simulink model "diff_drive"  (R2021b)
settings: Solver=VariableStepAuto  StartTime=0.0  StopTime=10.0  RelTol=1e-3
settings Model: Creator=Daniel  LastModifiedBy=Daniel

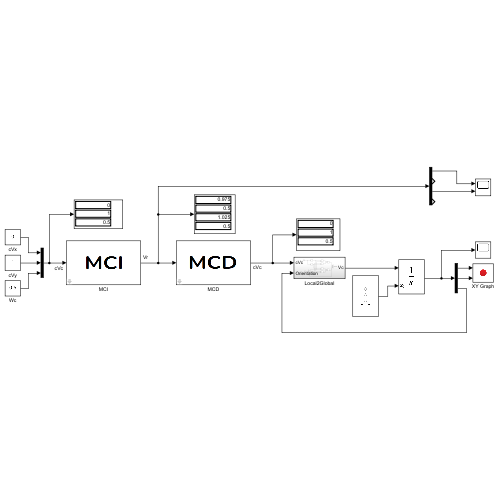
[thumbnail: Simulink's stored preview of the top-level diagram]
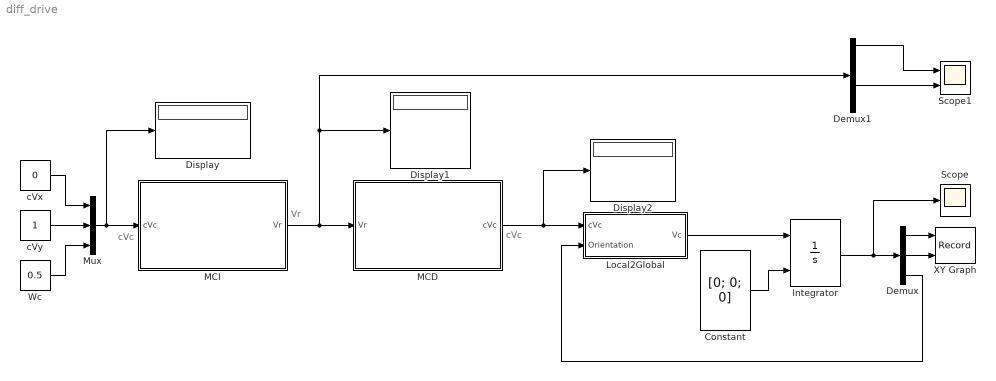
== system diff_drive ==
  note: cVc
  note: Vr
  note: cVc
  Constant : Constant  Value=[0; 0; 0]  VectorParams1D=off  SampleTime=-1
  Demux : Demux  Outputs=3
  Demux1 : Demux
  Display : Display
  Display1 : Display
  Display2 : Display
  Integrator : Integrator  InitialConditionSource=external
  Local2Global : Subsystem
  MCD : Subsystem  mask{d1=0.05, d2=0.05}
      mask prompts: d1 "Distancia del centro a la rueda 1 (m)"; d2 "Distancia del centro a la rueda 1 (m)"
      mask Display: image('$imagefile'); % Use "Edit Image" on toolstrip to change.
  MCI : Subsystem  mask{d1=0.05, d2=0.05}
      mask prompts: d1 "Distancia del centro a la rueda 1 (m)"; d2 "Distancia del centro a la rueda 2 (m)"
      mask Display: image('$imagefile'); % Use "Edit Image" on toolstrip to change.
  Mux : Mux  Inputs=3
  Scope : Scope
  Scope1 : Scope  NumInputPorts=2
  Wc : Constant  Value=0.5
  XY Graph : Record  FileSettingsInternal="{\"entries\":[{\"content\":{\"excelSettings\":{\"content\":{},\"type\":\"Streamout.ExcelSettings\"}},\"type\":\"Streamout.FileSettingStorage\",\"uuid\":\"aee6dd4d-bbbd-48c0-9c27-9c7c50ef588e\"}],\"packageUris\":[\"http://schema.mathworks.com/mf0/streamout_blocks/R2020a\"],\"version\":\"1.0\"}"  Layout=[1 1]  SignalsInternal="{\"entries\":[{\"content\":{\"signals\":[{\"content\":{\"blockPath\":[\"diff_drive/XY Graph\"],\"channel\":[],\"dimensions\":[1,1],\"domain\":\"diff_drive/XY Graph\",\"lineColor\":\"#a2142f\",\"plots\":[1],\"port\":1,\"sid\":[\"\"],\"signalID\":20,\"signalName\":\"Demux:1\"},\"type\":\"RecordBlkView.Signal\",\"uuid\":\"20fe10e5-6b37-4d22-ab0f-be3f28a80425\"},{\"content\":{\"blockPath\":[\"diff_drive/XY Graph\"],\"channel\":[],\"dimensions\":[1,1],\"domain\":\"diff_drive/XY Graph\",\"lineColor\":\"#139fff\",\"plots\":[1],\"port\":2,\"sid\":[\"\"],\"signalID\":24,\"signalName\":\"Demux:2\"},\"type\":\"RecordBlkView.Signal\",\"uuid\":\"9389c952-68ea-4058-aac4-d4c33f5d623a\"}]},\"type\":\"RecordBlkView.InputSignals\",\"uuid\":\"ce8dd289-cd3d-4bba-880f-7e18354d1495\"}],\"packageUris\":[\"http://schema.mathworks.com/mf0/streamout_blocks/R2020a\"],\"version\":\"1.0\"}"  VisualizationBindings="{\"xyplotplugin\":{\"info\":[{\"series\":[{\"bindingParametersList\":[{\"parameter\":\"X-Axis\",\"signalID\":20,\"signalName\":\"Demux:1\"},{\"parameter\":\"Y-Axis\",\"signalID\":24,\"signalName\":\"Demux:2\"}],\"seriesID\":39278}],\"subplotID\":1}]}}"  CompatibilityTag=XY
  cVx : Constant  Value=0
  cVy : Constant
  wires:
  Mux/1 -> Display/1, MCI/1(cVc)
  cVy/1 -> Mux/2
  cVx/1 -> Mux/1
  Wc/1 -> Mux/3
  Constant/1 -> Integrator/2
  Integrator/1 -> Demux/1, Scope/1
  Demux/1 -> XY Graph/1
  Demux/2 -> XY Graph/2
  MCI/1(Vr) -> Demux1/1, Display1/1, MCD/1(Vr)
  MCD/1(cVc) -> Display2/1, Local2Global/1(cVc)
  Local2Global/1(Vc) -> Integrator/1
  Demux/3 -> Local2Global/2(Orientation)
  Demux1/1 -> Scope1/1
  Demux1/3 -> Scope1/2

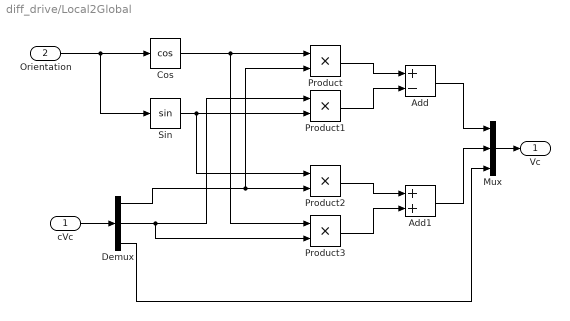
== system diff_drive/Local2Global ==
  cVc : Inport
  Orientation : Inport  Port=2
  Add : Sum  Inputs=+-
  Add1 : Sum
  Cos : Trigonometry  Operator=cos
  Demux : Demux  Outputs=3
  Mux : Mux  Inputs=3
  Product{,1..3} (4 alike) : Product
  Sin : Trigonometry
  Vc : Outport
  wires:
  Orientation/1 -> Sin/1, Cos/1
  cVc/1 -> Demux/1
  Cos/1 -> Product3/1, Product/1
  Demux/1 -> Product/2, Product2/2
  Product/1 -> Add/1
  Product2/1 -> Add1/1
  Product3/1 -> Add1/2
  Demux/2 -> Product3/2, Product1/1
  Sin/1 -> Product2/1, Product1/2
  Mux/1 -> Vc/1
  Add/1 -> Mux/1
  Add1/1 -> Mux/2
  Demux/3 -> Mux/3
  Product1/1 -> Add/2

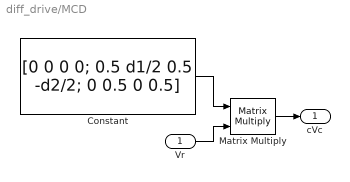
== system diff_drive/MCD ==
  Vr : Inport
  Constant : Constant  Value=[0 0 0 0; 0.5 d1/2 0.5 -d2/2; 0 0.5 0 0.5]  VectorParams1D=off
  Matrix Multiply : Product  Multiplication=Matrix(*)
  cVc : Outport
  wires:
  Matrix Multiply/1 -> cVc/1
  Vr/1 -> Matrix Multiply/2
  Constant/1 -> Matrix Multiply/1

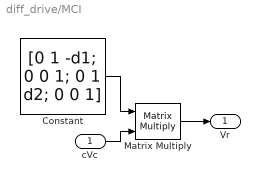
== system diff_drive/MCI ==
  cVc : Inport
  Constant : Constant  Value=[0 1 -d1; 0 0 1; 0 1 d2; 0 0 1]  VectorParams1D=off
  Matrix Multiply : Product  Multiplication=Matrix(*)
  Vr : Outport
  wires:
  Matrix Multiply/1 -> Vr/1
  cVc/1 -> Matrix Multiply/2
  Constant/1 -> Matrix Multiply/1
